simulink model "visualization"  (R2021b)
settings: Solver=VariableStepAuto  StartTime=0.0  StopTime=34  RelTol=1e-3
libraries: sharedtransform x1, sim3dcameralib x1, sim3dlib x1, uavsim3dlib x1
settings Model: Creator=matthew  LastModifiedBy=matthew

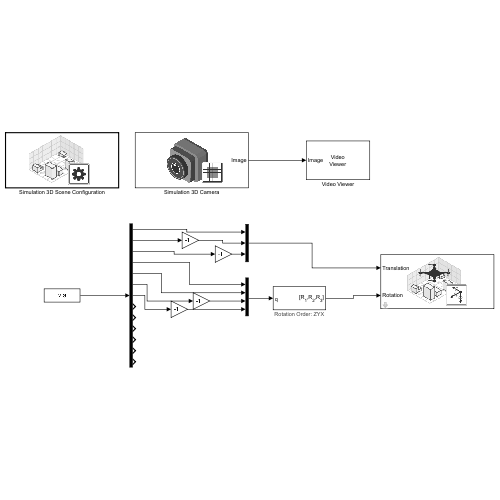
[thumbnail: Simulink's stored preview of the top-level diagram]
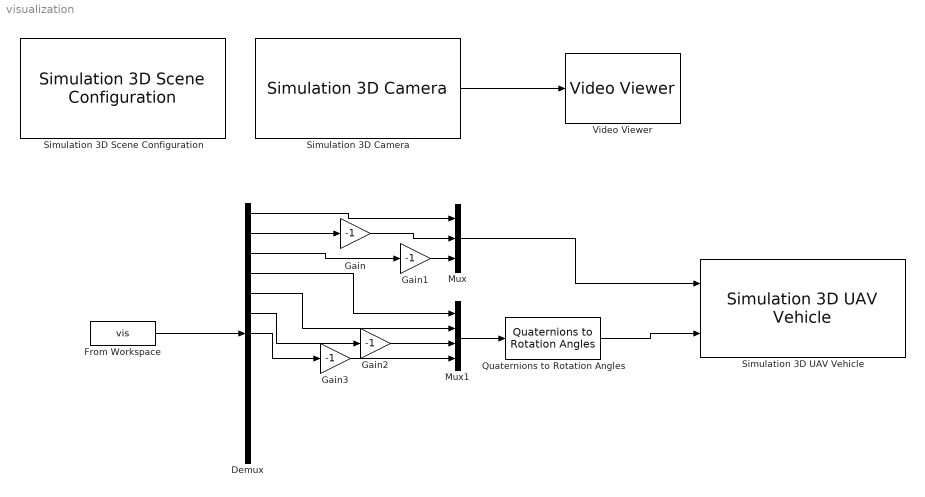
== system visualization ==
  Demux : Demux  Outputs=13
  From Workspace : FromWorkspace  VariableName=vis
  Gain{,1..3} (4 alike) : Gain  Gain=-1
  Mux : Mux  Inputs=3
  Mux1 : Mux
  Quaternions to Rotation Angles : sharedtransform/Quaternions to Rotation Angles  rotationOrder=ZYX  aMode=aMode
      settings: SourceProductBaseCode=AE,PW,DR,MT,UV,VE
  Simulation 3D Camera : sim3dcameralib/Simulation 3D Camera  Priority=1  sensorTag=Sim3dSensor1  sensorId=1  sensorName=Sim3dSensor1  vehTagList={'Scene Origin';'heli1'}  vehTag=heli1  mountLoc=Origin  offsetFlag=on  tmountOffset=[-3, 0, 0]  extTmount=off  rmountOffset=[0, 0, 0]  extRmount=off  FocalLength=[1109, 1109]  OpticalCenter=[640, 360]  ImageSize=[720, 1280]  RadialDistortion=[0, 0]  TangentialDistortion=[0, 0]  SensorSkew=0  DepthOutportEnabled=off  SemanticOutportEnabled=off  TransformOutportEnabled=off  SampleTime=-1  mountPoint=[-3 0 0]  mountOrientation=[0 0 0]  aMode=4  ID=1
      settings: SourceProductBaseCode=AE,DR,UV,VE
  Simulation 3D Scene Configuration : sim3dlib/Simulation 3D Scene Configuration  Priority=0  ProjectFormat_internal=Default Scenes  ProjectFormat=Default Scenes  SceneDesc=US city block  ProjectName=W:\R2021b\toolbox\shared\sim3d_projects\automotive_project\UE4\WindowsNoEditor\VehicleSimulation.exe  ScenePath=/Game/Maps/USCityBlock  vehTagList={'Scene Origin';'heli1'}  vehTag=heli1  OpVisEn=off  Ts=1/60  EnableWindow=on  EnableWeather=off  SunAltitude=40.0  SunAzimuth=90  clouds=10  wind=1  fog=0  rain=0  sensorTag=MainCamera1  sensorId=1  sensorName=MainCamera1  mountLoc=Origin  offsetFlag=off  tmountOffset=[0, 0, 0]  rmountOffset=[0, 0, 0]  HorizontalResolution=1280  VerticalResolution=720  HorizontalFOV=60  mountPoint=[0 0 0]  mountOrientation=[0 0 0]  aMode=4  ID=1
      settings: SourceProductBaseCode=AE,DR,UV,VE
  Simulation 3D UAV Vehicle : uavsim3dlib/Simulation 3D UAV Vehicle  Priority=-1  Mesh=Quadrotor  MeshPath=/MathWorksUAVContent/UAVs/HexaRotorUAV/HexaRotor.HexaRotor  Color=Black  ActorName=heli1  InitialTranslation=[0 0 0]  InitialRotation=[0 0 0]  SampleTime=-1  ActorType=SimulinkVehicle  ID=C  aMode=4  ActorTag=heli1
      settings: SourceProductBaseCode=UV
  Video Viewer : VideoViewer  FigPos=[795 900 1017 607]
  wires:
  From Workspace/1 -> Demux/1
  Simulation 3D Camera/1 -> Video Viewer/1
  Mux/1 -> Simulation 3D UAV Vehicle/1
  Demux/1 -> Mux/1
  Demux/4 -> Mux1/1
  Demux/5 -> Mux1/2
  Demux/6 -> Gain2/1
  Demux/7 -> Gain3/1
  Mux1/1 -> Quaternions to Rotation Angles/1
  Quaternions to Rotation Angles/1 -> Simulation 3D UAV Vehicle/2
  Demux/2 -> Gain/1
  Gain/1 -> Mux/2
  Gain1/1 -> Mux/3
  Demux/3 -> Gain1/1
  Gain2/1 -> Mux1/3
  Gain3/1 -> Mux1/4
